simulink model "water_4hopper_VDF"  (Simulink 8.0)
settings: Solver=ode23t  StartTime=0.0  StopTime=5  MaxStep=1e-2  RelTol=1e-6
values from neighbouring files (symbols this model uses):
  alpha = 30    [SimParam_4VDF.m]
  amp = leg_length    (= 0.0249)    [SimParam_4VDF.m]
  C_d = 0.703    [SimParam_4VDF.m]
  density = 1000    [SimParam_4VDF.m]
  frame_inertia = diag([Ix,Iy,Iz])    [SimParam_4VDF.m]
  freq = 60    [SimParam_4VDF.m]
  g = 9.81    [SimParam_4VDF.m]
  K_d = 0    [SimParam_4VDF.m]
  K_i = 0    [SimParam_4VDF.m]
  K_p = -50    [SimParam_4VDF.m]
  leg_length = 0.0249    [SimParam_4VDF.m]
  m_toe = 0.0    (= 0)    [SimParam_4VDF.m]
  mass = 0.1    [SimParam_4VDF.m]
  S1 = pi*r1^2*0.9185    (= 0.00115422114093)    [SimParam_4VDF.m]
  S2 = pi*r2^2*0.9185    (= 7.21388213081e-05)    [SimParam_4VDF.m]
  tau = 0.001    [SimParam_4VDF.m]
undefined symbols (not defined in the file): y_0
libraries: mblibv1 x48, powerlib_extras x4, simulink x2
(part 1 of 2)
settings Model: Creator=Metti  LastModifiedBy=Metti
settings SolverCC: ZeroCrossControl=DisableAll
settings DataIOCC: SignalLoggingSaveFormat=ModelDataLogs
settings DebuggingCC: FcnCallInpInsideContextMsg=EnableAllAsWarning
settings SimMechanicsCC: VisOnUpdateDiagram=on  VisDuringSimulation=on  VisSampleTime=0.05  AutoFitVis=GROWTOFIT  LastVizWinPosition=[520 378 560 420]  CamPosition=[0;0;11.3949;]  CamTarget=[0;0;0;]  CamUpVector=[0;1;0;]  CamHeight=0.51  VisBackgroundColor=[0.9;0.9;0.95;]  DefaultBodyColor=[1;0;0;]
settings ConfigurationSet: Description=SimMechanics 2G

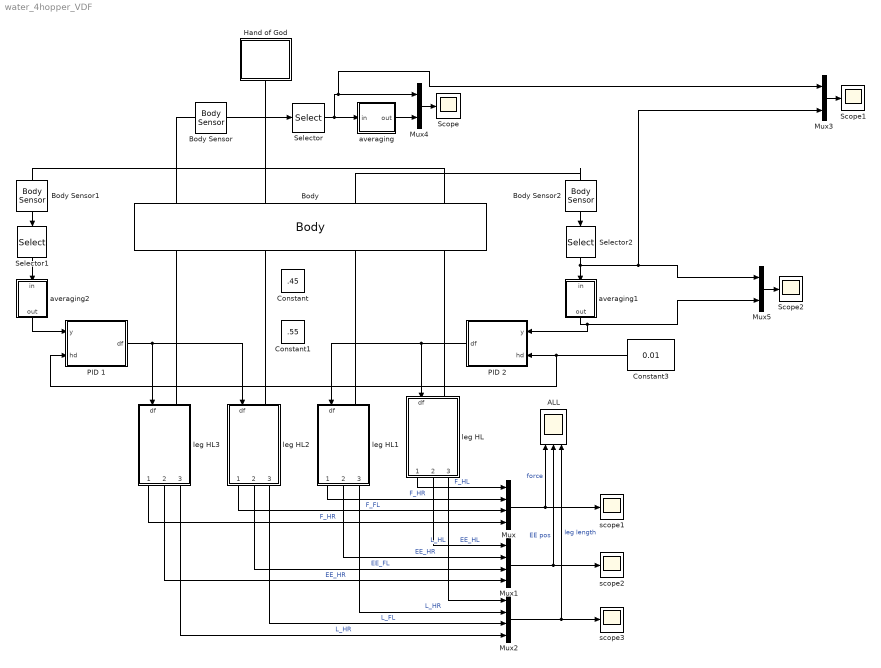
== system water_4hopper_VDF ==
  ALL : Scope  NumInputPorts=3
      settings: ShowLegends=on  TimeRange=10  YMin=-1~-50~-0.06  YMax=7~200~0.06  SaveName=ScopeData4
  Body : mblibv1/Bodies/Body  LConnTagsString=CG|CS1|CS6|CS7  RConnTagsString=CS2|CS3|CS4|CS5  UpdateFromCAD=off  DialogClass=MechanicalBodyBlock  Mass=mass  MassUnits=kg  InertiaUnits=kg*m^2  Inertia=frame_inertia  Shape=Cylinder  ShapeDims=[1 1]  ShapeUnits=m  ShapeUse=false  Density=1  DensityUnits=kg/m^3  DensityUse=false  GraphicsMode=MACHINE_DEFAULT  BodyColorSelMode=MACHINE_DEFAULT  BodyColor=[1 0 0]  AttachedToCS=CG  CG=Left$CG$CG_pos$CS1$CS1$m$[0 0 0]$Euler X-Y-Z$deg$WORLD$true$none  WorkingFrames=Left$CS1$[0 0 0]$Adjoining$Adjoining$m$[0 0 0]$Euler X-Y-Z$deg$WORLD$true$none#Right$CS2$TR_FR$CS1$CS1$m$[0 0 0]$Euler X-Y-Z$deg$WORLD$true$none#Right$CS3$TR_FL$CS1$CS1$m$[0 0 0]$Euler X-Y-Z$deg$WORLD$true$none#Right$CS4$TR_HR$CS1$CS1$m$[0 0 0]$Euler X-Y-Z$deg$WORLD$true$none#Right$CS5$TR_HL$CS1$CS1$m$[0 0 0]$Euler X-Y-Z$deg$WORLD$true$none#Left$CS6$TR_HL$CS1$CS1$m$[0 0 0]$Euler X-Y-Z$deg$WORLD$true$none#Left$CS7$TR_FR$CS1$CS1$m$[0 0 0]$Euler X-Y-Z$deg$WORLD$true$none  CGPos=CG_pos  CGRot=[0 0 0]  CS0Pos=[]  CS0Rot=[]  CS1Pos=[0 0 0]  CS1Rot=[0 0 0]  CS2Pos=TR_FR  CS2Rot=[0 0 0]  CS3Pos=TR_FL  CS3Rot=[0 0 0]  CS4Pos=TR_HR  CS4Rot=[0 0 0]  CS5Pos=TR_HL  CS5Rot=[0 0 0]  CS6Pos=TR_HL  CS6Rot=[0 0 0]  CS7Pos=TR_FR  CS7Rot=[0 0 0]  CS8Pos=[]  CS8Rot=[]  CS9Pos=[]  CS9Rot=[]  CS10Pos=[]  CS10Rot=[]  CS11Pos=[]  CS11Rot=[]  CS12Pos=[]  CS12Rot=[]  CS13Pos=[]  CS13Rot=[]  CS14Pos=[]  CS14Rot=[]  CS15Pos=[]  CS15Rot=[]  CS16Pos=[]  CS16Rot=[]  CS17Pos=[]  CS17Rot=[]  CS18Pos=[]  CS18Rot=[]  CS19Pos=[]  CS19Rot=[]  CS20Pos=[]  CS20Rot=[]
  Body Sensor : mblibv1/Sensors &  Actuators/Body Sensor  UpdateFromCAD=off  PhysicalDomain=Mechanical  PortType=blob  Muxed=on  Pose=off  Angle=on  AngleUnits=deg  ArcVelocity=off  ArcVelocityUnits=deg/s  ArcAcceleration=off  ArcAccelerationUnits=deg/s^2  CoordPosition=on  CoordPositionUnits=m  Velocity=off  VelocityUnits=m/s  Acceleration=off  AccelerationUnits=m/s^2  Quaternion=on  QuaternionDT=off  QuaternionDDT=off  QuaternionUnits=off  OutputVector=[1]  ActiveIO=on  Width=3  DialogClass=MechanicalSensorBlock  ReferenceFrame=Absolute (World)
  Body Sensor1 : mblibv1/Sensors &  Actuators/Body Sensor  UpdateFromCAD=off  PhysicalDomain=Mechanical  PortType=blob  Muxed=on  Pose=off  Angle=on  AngleUnits=deg  ArcVelocity=off  ArcVelocityUnits=deg/s  ArcAcceleration=off  ArcAccelerationUnits=deg/s^2  CoordPosition=on  CoordPositionUnits=m  Velocity=off  VelocityUnits=m/s  Acceleration=off  AccelerationUnits=m/s^2  Quaternion=on  QuaternionDT=off  QuaternionDDT=off  QuaternionUnits=off  OutputVector=[1]  ActiveIO=on  Width=3  DialogClass=MechanicalSensorBlock  ReferenceFrame=Absolute (World)
  Body Sensor2 : mblibv1/Sensors &  Actuators/Body Sensor  UpdateFromCAD=off  PhysicalDomain=Mechanical  PortType=blob  Muxed=on  Pose=off  Angle=on  AngleUnits=deg  ArcVelocity=off  ArcVelocityUnits=deg/s  ArcAcceleration=off  ArcAccelerationUnits=deg/s^2  CoordPosition=on  CoordPositionUnits=m  Velocity=off  VelocityUnits=m/s  Acceleration=off  AccelerationUnits=m/s^2  Quaternion=on  QuaternionDT=off  QuaternionDDT=off  QuaternionUnits=off  OutputVector=[1]  ActiveIO=on  Width=3  DialogClass=MechanicalSensorBlock  ReferenceFrame=Absolute (World)
  Constant : Constant  Value=.45
  Constant1 : Constant  Value=.55
  Constant3 : Constant  Value=0.01
  Hand of God : Subsystem
  Mux : Mux
  Mux1 : Mux
  Mux2 : Mux
  Mux3 : Mux  Inputs=2
  Mux4 : Mux  Inputs=2
  Mux5 : Mux  Inputs=2
  PID 1 : Subsystem
  PID 2 : Subsystem
  Scope : Scope
      settings: TimeRange=5  YMin=-0.025  YMax=0.02
  Scope1 : Scope
      settings: YMin=0.0915  YMax=0.09575  SaveName=ScopeData5
  Scope2 : Scope
      settings: YMin=0.0915  YMax=0.09575  SaveName=ScopeData12
  Selector : Selector  InputPortWidth=3  IndexOptions=Index vector (dialog)  Indices=[2]  OutputSizes=1
  Selector1 : Selector  InputPortWidth=3  IndexOptions=Index vector (dialog)  Indices=[2]  OutputSizes=1
  Selector2 : Selector  InputPortWidth=3  IndexOptions=Index vector (dialog)  Indices=[2]  OutputSizes=1
  averaging : Subsystem  mask{T_win=2*pi/freq/2, x_init=y_0}
      mask prompts: T_win "window (s)"; x_init "Initial condition"
  averaging1 : Subsystem  mask{T_win=2*pi/freq, x_init=y_0}
      mask prompts: T_win "window (s)"; x_init "Initial condition"
  averaging2 : Subsystem  mask{T_win=2*pi/freq, x_init=y_0}
      mask prompts: T_win "window (s)"; x_init "Initial condition"
  leg HL : Subsystem
  leg HL1 : Subsystem
  leg HL2 : Subsystem
  leg HL3 : Subsystem
  "scope1 " : Scope
      settings: ShowLegends=on
  scope2 : Scope
      settings: ShowLegends=on  SaveName=ScopeData2
  scope3 : Scope
      settings: ShowLegends=on  SaveName=ScopeData3
  wires:
  Body Sensor/1 -> Selector/1
  Mux/1 -> "scope1 "/1, ALL/1  "force"
  leg HL/1(force) -> Mux/1  "F_HL"
  leg HL1/1(force) -> Mux/2  "F_HR"
  leg HL2/1(force) -> Mux/3  "F_FL"
  leg HL3/1(force) -> Mux/4  "F_HR"
  Mux1/1 -> ALL/2, scope2/1  "EE pos"
  leg HL/2(EE pos) -> Mux1/1  "EE_HL"
  leg HL1/2(EE pos) -> Mux1/2  "EE_HR"
  leg HL3/2(EE pos) -> Mux1/4  "EE_HR"
  leg HL2/2(EE pos) -> Mux1/3  "EE_FL"
  Mux2/1 -> ALL/3, scope3/1  "leg length"
  leg HL/3(leg length) -> Mux2/1  "L_HL"
  leg HL1/3(leg length) -> Mux2/2  "L_HR"
  leg HL2/3(leg length) -> Mux2/3  "L_FL"
  leg HL3/3(leg length) -> Mux2/4  "L_HR"
  averaging/1(out) -> Mux4/2
  Mux4/1 -> Scope/1
  Body Sensor1/1 -> Selector1/1
  Body Sensor2/1 -> Selector2/1
  Selector2/1 -> averaging1/1(in), Mux3/2, Mux5/1
  Constant3/1 -> PID 1/2(hd), PID 2/2(hd)
  Selector1/1 -> averaging2/1(in)
  Mux5/1 -> Scope2/1
  averaging1/1(out) -> PID 2/1(y), Mux5/2
  averaging2/1(out) -> PID 1/1(y)
  PID 2/1(df) -> leg HL1/1(df), leg HL/1(df)
  PID 1/1(df) -> leg HL3/1(df), leg HL2/1(df)
  Mux3/1 -> Scope1/1
  Selector/1 -> averaging/1(in), Mux3/1, Mux4/1
  connections:
  Hand of God/RConn1 -- Body/LConn2
  leg HL2/LConn1 -- Body/RConn2
  leg HL1/LConn1 -- Body/RConn3
  Body/RConn4 -- leg HL/LConn1
  leg HL3/LConn1 -- Body/RConn1
  Body Sensor1/LConn1 -- Body/LConn4
  Body Sensor2/LConn1 -- Body/LConn3
  Body Sensor/LConn1 -- Body/LConn1

== system water_4hopper_VDF/Hand of God ==
  Custom Joint : mblibv1/Joints/Custom Joint  LConnTagsString=__newl0|SA1  RConnTagsString=__newr0  UpdateFromCAD=off  NumSAPorts=1  CutJoint=off  MarkAsCut=off  Primitives=prismatic  PrimitiveProps=P1$World$[0 1 0]$Prismatic#P2$World$[1 0 0]$Prismatic#R1$World$[1 0 0]$Revolute#R2$World$[0 0 1]$Revolute  DialogClass=JointBlock  R1Axis=[1 0 0]  R2Axis=[0 0 1]  R3Axis=[]  P1Axis=[0 1 0]  P2Axis=[1 0 0]  P3Axis=[]  SAxis=[]
  Ground : mblibv1/Bodies/Ground  UpdateFromCAD=off  LeftPortType=env  RightPortType=workingframe  PhysicalDomain=Mechanical  DialogClass=GroundBlock  CoordPosition=[0 0 0]  CoordPositionUnits=m  StateVectorMgrId=0  MachineId=[1 0]  ShowEnvPort=on
  Joint Initial Condition : mblibv1/Sensors &  Actuators/Joint Initial Condition  UpdateFromCAD=off  LeftPortType=blob  RightPortType=blob  PhysicalDomain=mechanical  DialogClass=InitialConditionBlock  InitialConditions=P1$true$y_0$m$deg$0$m/s$deg/s#P2$false$y_0$m$deg$0$m/s$deg/s#P3$false$0$m$deg$0$m/s$deg/s#R1$true$0$m$deg$0$m/s$deg/s#R2$true$0$m$deg$0$m/s$deg/s#R3$false$10$m$deg$0$m/s$deg/s#S$false$0$m$deg$0$m/s$deg/s  P1PIC=y_0  P1VIC=0  P2PIC=0  P2VIC=0  P3PIC=0  P3VIC=0  R1PIC=0  R1VIC=0  R2PIC=0  R2VIC=0  R3PIC=0  R3VIC=0  SPIC=0  SVIC=0
  Joint Sensor : mblibv1/Sensors &  Actuators/Joint Sensor  UpdateFromCAD=off  PhysicalDomain=Mechanical  PortType=blob  Muxed=on  Pose=off  Angle=on  AngleUnits=deg  ArcVelocity=off  ArcVelocityUnits=deg/s  ArcAcceleration=off  ArcAccelerationUnits=deg/s^2  CoordPosition=on  CoordPositionUnits=m  Velocity=off  VelocityUnits=m/s  Acceleration=off  AccelerationUnits=m/s^2  Quaternion=on  QuaternionDT=off  QuaternionDDT=off  QuaternionUnits=off  OutputVector=[1]  ActiveIO=on  Width=1  DialogClass=MechanicalSensorBlock  Primitive=P1  Force=off  ForceUnits=N  Torque=off  TorqueUnits=N*m  ReferenceFrame=Absolute (World)  ReactionSensedSide=Base  ReactionReferenceFrame=Absolute (World)  ReactionForce=off  ReactionForceUnits=N  ReactionMoment=off  ReactionMomentUnits=N*m
  Joint Sensor1 : mblibv1/Sensors &  Actuators/Joint Sensor  UpdateFromCAD=off  PhysicalDomain=Mechanical  PortType=blob  Muxed=on  Pose=off  Angle=on  AngleUnits=deg  ArcVelocity=off  ArcVelocityUnits=deg/s  ArcAcceleration=off  ArcAccelerationUnits=deg/s^2  CoordPosition=on  CoordPositionUnits=m  Velocity=off  VelocityUnits=m/s  Acceleration=off  AccelerationUnits=m/s^2  Quaternion=on  QuaternionDT=off  QuaternionDDT=off  QuaternionUnits=off  OutputVector=[1]  ActiveIO=on  Width=1  DialogClass=MechanicalSensorBlock  Primitive=R1  Force=off  ForceUnits=N  Torque=off  TorqueUnits=N*m  ReferenceFrame=Absolute (World)  ReactionSensedSide=Base  ReactionReferenceFrame=Absolute (World)  ReactionForce=off  ReactionForceUnits=N  ReactionMoment=off  ReactionMomentUnits=N*m
  Joint Sensor2 : mblibv1/Sensors &  Actuators/Joint Sensor  UpdateFromCAD=off  PhysicalDomain=Mechanical  PortType=blob  Muxed=off  Pose=off  Angle=on  AngleUnits=deg  ArcVelocity=off  ArcVelocityUnits=deg/s  ArcAcceleration=off  ArcAccelerationUnits=deg/s^2  CoordPosition=on  CoordPositionUnits=m  Velocity=off  VelocityUnits=m/s  Acceleration=off  AccelerationUnits=m/s^2  Quaternion=on  QuaternionDT=off  QuaternionDDT=off  QuaternionUnits=off  OutputVector=[1]  ActiveIO=on  Width=1  DialogClass=MechanicalSensorBlock  Primitive=R2  Force=off  ForceUnits=N  Torque=off  TorqueUnits=N*m  ReferenceFrame=Absolute (World)  ReactionSensedSide=Base  ReactionReferenceFrame=Absolute (World)  ReactionForce=off  ReactionForceUnits=N  ReactionMoment=off  ReactionMomentUnits=N*m
  Machine Environment : mblibv1/Bodies/Machine Environment  PortType=env  PhysicalDomain=Mechanical  DialogTemplateClass=MECH.MachineEnvironment  SyncWhenCopied=off  Gravity=[0 -g 0]  GravityUnits=m/s^2  GravityAsSignal=off  Dimensionality=Auto-detect  AnalysisType=Forward dynamics  LinearAssemblyTolerance=1e-3  LinearAssemblyToleranceUnits=m  AngularAssemblyTolerance=1e-3  AngularAssemblyToleranceUnits=rad  ConstraintSolverType=Stabilizing  ConstraintRelTolerance=1e-4  ConstraintAbsTolerance=1e-4  UseRobustSingularityHandling=off  RedundancyAnalysisToleranceType=Automatically select tolerance  RedundancyAnalysisTolerance=1e-14  StatePerturbationType=Fixed  PerturbationSize=1e-5  VisualizeMachine=on  BodyVisualizationType=Use model default body geometries  BodyColorSelMode=Use model default  DefaultBodyColor=[1 0 0]
  Mechanical Branching Bar : mblibv1/Utilities/Mechanical Branching Bar  LConnTagsString=_newl0  RConnTagsString=__newr0|SA2|SA3|SA4  UpdateFromCAD=off  DialogClass=MechanicalBranchingBarBlock  NumSAPorts=4
  Scope : Scope  NumInputPorts=3
      settings: TimeRange=5  YMin=-0.01~-0.001~-6  YMax=0.02~0.0004~1  SaveName=mass_data
  Conn1 : PMIOPort  Port=1  Side=Right
  wires:
  Joint Sensor/1 -> Scope/1
  Joint Sensor1/1 -> Scope/2
  Joint Sensor2/1 -> Scope/3
  connections:
  Conn1/RConn1 -- Custom Joint/RConn1
  Joint Sensor1/LConn1 -- Mechanical Branching Bar/RConn3
  Ground/RConn1 -- Custom Joint/LConn1
  Machine Environment/RConn1 -- Ground/LConn1
  Joint Initial Condition/RConn1 -- Mechanical Branching Bar/RConn1
  Joint Sensor/LConn1 -- Mechanical Branching Bar/RConn2
  Custom Joint/LConn2 -- Mechanical Branching Bar/LConn1
  Joint Sensor2/LConn1 -- Mechanical Branching Bar/RConn4

== system water_4hopper_VDF/PID 1 ==
  y : Inport
  hd : Inport  Port=2
  Constant : Constant  Value=.55
  Fcn : Fcn  Expr=u(1)^2
  Fcn1 : Fcn  Expr=u(1)^2
  Gain3 : Gain
  Mux4 : Mux  Inputs=2
  PID Controller : simulink/Continuous/PID Controller  Controller=PID  TimeDomain=Continuous-time  SampleTime=1  IntegratorMethod=Forward Euler  FilterMethod=Forward Euler  Form=Parallel  P=K_p  I=K_i  D=K_d  N=100  InitialConditionSource=internal  InitialConditionForIntegrator=0  InitialConditionForFilter=0  ExternalReset=none  LimitOutput=off  UpperSaturationLimit=inf  LowerSaturationLimit=-inf  LinearizeAsGain=on  AntiWindupMode=none  Kb=1  TrackingMode=off  Kt=1  PParamMin=[]  PParamMax=[]  IParamMin=[]  IParamMax=[]  DParamMin=[]  DParamMax=[]  NParamMin=[]  NParamMax=[]  KbParamMin=[]  KbParamMax=[]  KtParamMin=[]  KtParamMax=[]  POutMin=[]  POutMax=[]  IOutMin=[]  IOutMax=[]  DOutMin=[]  DOutMax=[]  NOutMin=[]  NOutMax=[]  KbOutMin=[]  KbOutMax=[]  KtOutMin=[]  KtOutMax=[]  IntegratorOutMin=[]  IntegratorOutMax=[]  FilterOutMin=[]  FilterOutMax=[]  SumOutMin=[]  SumOutMax=[]  SumI1OutMin=[]  SumI1OutMax=[]  SumI2OutMin=[]  SumI2OutMax=[]  SumI3OutMin=[]  SumI3OutMax=[]  SumDOutMin=[]  SumDOutMax=[]  SaturationOutMin=[]  SaturationOutMax=[]  IntegratorContinuousStateAttributes=''  IntegratorStateMustResolveToSignalObject=off  IntegratorRTWStateStorageClass=Auto  FilterContinuousStateAttributes=''  FilterStateMustResolveToSignalObject=off  FilterRTWStateStorageClass=Auto
  Saturation2 : Saturate  UpperLimit=0.7  LowerLimit=0.3
  Scope1 : Scope  NumInputPorts=2
      settings: TimeRange=5  YMin=0.0575~-0.0125  YMax=0.0875~0.015
  Scope3 : Scope
      settings: SaveName=ScopeData4
  Sum3 : Sum  Inputs=|+-
  Sum4 : Sum  Inputs=|-+
  df : Outport
  wires:
  PID Controller/1 -> Gain3/1
  Sum3/1 -> PID Controller/1, Scope1/2
  Gain3/1 -> Sum4/1
  Mux4/1 -> Scope1/1
  y/1 -> Fcn1/1, Mux4/2
  hd/1 -> Mux4/1, Fcn/1
  Sum4/1 -> Saturation2/1
  Saturation2/1 -> Scope3/1, df/1
  Constant/1 -> Sum4/2
  Fcn/1 -> Sum3/1
  Fcn1/1 -> Sum3/2

== system water_4hopper_VDF/PID 2 ==
  y : Inport
  hd : Inport  Port=2
  Constant : Constant  Value=.45
  Fcn : Fcn  Expr=u(1)^2
  Fcn1 : Fcn  Expr=u(1)^2
  Gain3 : Gain
  Mux4 : Mux  Inputs=2
  PID Controller : simulink/Continuous/PID Controller  Controller=PID  TimeDomain=Continuous-time  SampleTime=1  IntegratorMethod=Forward Euler  FilterMethod=Forward Euler  Form=Parallel  P=K_p  I=K_i  D=K_d  N=100  InitialConditionSource=internal  InitialConditionForIntegrator=0  InitialConditionForFilter=0  ExternalReset=none  LimitOutput=off  UpperSaturationLimit=inf  LowerSaturationLimit=-inf  LinearizeAsGain=on  AntiWindupMode=none  Kb=1  TrackingMode=off  Kt=1  PParamMin=[]  PParamMax=[]  IParamMin=[]  IParamMax=[]  DParamMin=[]  DParamMax=[]  NParamMin=[]  NParamMax=[]  KbParamMin=[]  KbParamMax=[]  KtParamMin=[]  KtParamMax=[]  POutMin=[]  POutMax=[]  IOutMin=[]  IOutMax=[]  DOutMin=[]  DOutMax=[]  NOutMin=[]  NOutMax=[]  KbOutMin=[]  KbOutMax=[]  KtOutMin=[]  KtOutMax=[]  IntegratorOutMin=[]  IntegratorOutMax=[]  FilterOutMin=[]  FilterOutMax=[]  SumOutMin=[]  SumOutMax=[]  SumI1OutMin=[]  SumI1OutMax=[]  SumI2OutMin=[]  SumI2OutMax=[]  SumI3OutMin=[]  SumI3OutMax=[]  SumDOutMin=[]  SumDOutMax=[]  SaturationOutMin=[]  SaturationOutMax=[]  IntegratorContinuousStateAttributes=''  IntegratorStateMustResolveToSignalObject=off  IntegratorRTWStateStorageClass=Auto  FilterContinuousStateAttributes=''  FilterStateMustResolveToSignalObject=off  FilterRTWStateStorageClass=Auto
  Saturation2 : Saturate  UpperLimit=0.7  LowerLimit=0.3
  Scope1 : Scope  NumInputPorts=2
      settings: TimeRange=5  YMin=0.0575~-0.0125  YMax=0.0875~0.015
  Scope3 : Scope
      settings: SaveName=ScopeData4
  Sum3 : Sum  Inputs=|+-
  Sum4 : Sum  Inputs=|-+
  df : Outport
  wires:
  PID Controller/1 -> Gain3/1
  Sum3/1 -> Scope1/2, PID Controller/1
  Gain3/1 -> Sum4/1
  Mux4/1 -> Scope1/1
  Sum4/1 -> Saturation2/1
  Constant/1 -> Sum4/2
  Fcn/1 -> Sum3/1
  Fcn1/1 -> Sum3/2
  y/1 -> Fcn1/1, Mux4/2
  hd/1 -> Mux4/1, Fcn/1
  Saturation2/1 -> Scope3/1, df/1

== system water_4hopper_VDF/averaging ==
  in : Inport
  Constant1 : Constant  Value=x_init
  Gain : Gain  Gain=1/T_win
  Integrator1 : Integrator
  Sum : Sum  Inputs=+-|
  Sum1 : Sum  Inputs=-+|
  Sum3 : Sum  Inputs=++|
  Transport Delay : TransportDelay  DelayTime=T_win
  out : Outport
  wires:
  in/1 -> Sum1/2
  Gain/1 -> Sum3/2
  Constant1/1 -> Sum3/1, Sum1/1
  Sum1/1 -> Integrator1/1
  Transport Delay/1 -> Sum/2
  Integrator1/1 -> Sum/1, Transport Delay/1
  Sum3/1 -> out/1
  Sum/1 -> Gain/1

== system water_4hopper_VDF/averaging1 ==
  in : Inport
  Constant1 : Constant  Value=x_init
  Gain : Gain  Gain=1/T_win
  Integrator1 : Integrator
  Sum : Sum  Inputs=+-|
  Sum1 : Sum  Inputs=-+|
  Sum3 : Sum  Inputs=++|
  Transport Delay : TransportDelay  DelayTime=T_win
  out : Outport
  wires:
  in/1 -> Sum1/2
  Gain/1 -> Sum3/2
  Constant1/1 -> Sum3/1, Sum1/1
  Sum1/1 -> Integrator1/1
  Transport Delay/1 -> Sum/2
  Integrator1/1 -> Sum/1, Transport Delay/1
  Sum3/1 -> out/1
  Sum/1 -> Gain/1

== system water_4hopper_VDF/averaging2 ==
  in : Inport
  Constant1 : Constant  Value=x_init
  Gain : Gain  Gain=1/T_win
  Integrator1 : Integrator
  Sum : Sum  Inputs=+-|
  Sum1 : Sum  Inputs=-+|
  Sum3 : Sum  Inputs=++|
  Transport Delay : TransportDelay  DelayTime=T_win
  out : Outport
  wires:
  Sum/1 -> Gain/1
  Sum3/1 -> out/1
  Integrator1/1 -> Transport Delay/1, Sum/1
  Transport Delay/1 -> Sum/2
  Sum1/1 -> Integrator1/1
  Constant1/1 -> Sum1/1, Sum3/1
  Gain/1 -> Sum3/2
  in/1 -> Sum1/2

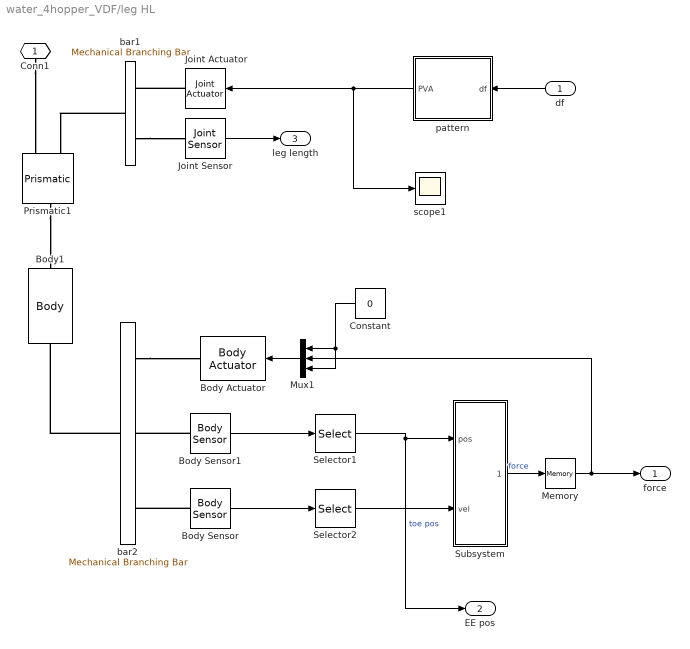
== system water_4hopper_VDF/leg HL ==
  df : Inport
  Body Actuator : mblibv1/Sensors &  Actuators/Body Actuator  UpdateFromCAD=off  PhysicalDomain=Mechanical  PortType=blob  ActuationStyle=Force  AngleUnits=deg  ArcVelocityUnits=deg/s  ArcAccelerationUnits=deg/s^2  CoordPositionUnits=m  VelocityUnits=m/s  AccelerationUnits=m/s^2  ForceUnits=N  TorqueUnits=N*m  ActiveIO=on  Width=3  DialogClass=MechanicalActuatorBlock  ReferenceFrame=Local (Body CS)  Angle=off  CoordPosition=on  Force=on  Torque=off
  Body Sensor : mblibv1/Sensors &  Actuators/Body Sensor  UpdateFromCAD=off  PhysicalDomain=Mechanical  PortType=blob  Muxed=on  Pose=off  Angle=on  AngleUnits=deg  ArcVelocity=off  ArcVelocityUnits=deg/s  ArcAcceleration=off  ArcAccelerationUnits=deg/s^2  CoordPosition=off  CoordPositionUnits=m  Velocity=on  VelocityUnits=m/s  Acceleration=off  AccelerationUnits=m/s^2  Quaternion=on  QuaternionDT=off  QuaternionDDT=off  QuaternionUnits=off  OutputVector=[1]  ActiveIO=on  Width=3  DialogClass=MechanicalSensorBlock  ReferenceFrame=Local (Body CS)
  Body Sensor1 : mblibv1/Sensors &  Actuators/Body Sensor  UpdateFromCAD=off  PhysicalDomain=Mechanical  PortType=blob  Muxed=on  Pose=off  Angle=on  AngleUnits=deg  ArcVelocity=off  ArcVelocityUnits=deg/s  ArcAcceleration=off  ArcAccelerationUnits=deg/s^2  CoordPosition=on  CoordPositionUnits=m  Velocity=off  VelocityUnits=m/s  Acceleration=off  AccelerationUnits=m/s^2  Quaternion=on  QuaternionDT=off  QuaternionDDT=off  QuaternionUnits=off  OutputVector=[1]  ActiveIO=on  Width=3  DialogClass=MechanicalSensorBlock  ReferenceFrame=Absolute (World)
  Body1 : mblibv1/Bodies/Body  LConnTagsString=CG  RConnTagsString=CS1  UpdateFromCAD=off  DialogClass=MechanicalBodyBlock  Mass=m_toe  MassUnits=kg  InertiaUnits=kg*m^2  Inertia=0.*eye(3)  Shape=Cylinder  ShapeDims=[1 1]  ShapeUnits=m  ShapeUse=false  Density=1  DensityUnits=kg/m^3  DensityUse=false  GraphicsMode=CONVHULL  BodyColorSelMode=MACHINE_DEFAULT  BodyColor=[1 0 0]  AttachedToCS=CG  CG=Left$CG$[0 0 0]$Adjoining$Adjoining$m$[0 0 0]$Euler X-Y-Z$deg$WORLD$true$none  WorkingFrames=Right$CS1$[0 -leg_length 0]$CG$CG$m$[0 0 0]$Euler X-Y-Z$deg$WORLD$true$none#Left$CS2$[0 0 0]$CG$CG$m$[0 0 0]$Euler X-Y-Z$deg$WORLD$false$none  CGPos=[0 0 0]  CGRot=[0 0 0]  CS0Pos=[]  CS0Rot=[]  CS1Pos=[0 -leg_length 0]  CS1Rot=[0 0 0]  CS2Pos=[0 0 0]  CS2Rot=[0 0 0]  CS3Pos=[]  CS3Rot=[]  CS4Pos=[]  CS4Rot=[]  CS5Pos=[]  CS5Rot=[]  CS6Pos=[]  CS6Rot=[]  CS7Pos=[]  CS7Rot=[]  CS8Pos=[]  CS8Rot=[]  CS9Pos=[]  CS9Rot=[]  CS10Pos=[]  CS10Rot=[]  CS11Pos=[]  CS11Rot=[]  CS12Pos=[]  CS12Rot=[]  CS13Pos=[]  CS13Rot=[]  CS14Pos=[]  CS14Rot=[]  CS15Pos=[]  CS15Rot=[]  CS16Pos=[]  CS16Rot=[]  CS17Pos=[]  CS17Rot=[]  CS18Pos=[]  CS18Rot=[]  CS19Pos=[]  CS19Rot=[]  CS20Pos=[]  CS20Rot=[]
  Constant : Constant  Value=0
  Joint Actuator : mblibv1/Sensors &  Actuators/Joint Actuator  UpdateFromCAD=off  PhysicalDomain=Mechanical  PortType=blob  ActuationStyle=Motion  AngleUnits=deg  ArcVelocityUnits=deg/s  ArcAccelerationUnits=deg/s^2  CoordPositionUnits=m  VelocityUnits=m/s  AccelerationUnits=m/s^2  ForceUnits=N  TorqueUnits=N*m  ActiveIO=on  Width=3  DialogClass=MechanicalActuatorBlock  Primitive=P1  ReferenceFrame=Absolute (World)
  Joint Sensor : mblibv1/Sensors &  Actuators/Joint Sensor  UpdateFromCAD=off  PhysicalDomain=Mechanical  PortType=blob  Muxed=on  Pose=off  Angle=on  AngleUnits=deg  ArcVelocity=off  ArcVelocityUnits=deg/s  ArcAcceleration=off  ArcAccelerationUnits=deg/s^2  CoordPosition=on  CoordPositionUnits=m  Velocity=off  VelocityUnits=m/s  Acceleration=off  AccelerationUnits=m/s^2  Quaternion=on  QuaternionDT=off  QuaternionDDT=off  QuaternionUnits=off  OutputVector=[1]  ActiveIO=on  Width=1  DialogClass=MechanicalSensorBlock  Primitive=P1  Force=off  ForceUnits=N  Torque=off  TorqueUnits=N*m  ReferenceFrame=Absolute (World)  ReactionSensedSide=Base  ReactionReferenceFrame=Absolute (World)  ReactionForce=off  ReactionForceUnits=N  ReactionMoment=off  ReactionMomentUnits=N*m
  Memory : Memory
  Mux1 : Mux  Inputs=3
  Prismatic1 : mblibv1/Joints/Prismatic  LConnTagsString=__newl0|SA1  RConnTagsString=__newr0  UpdateFromCAD=off  NumSAPorts=1  CutJoint=off  MarkAsCut=off  Primitives=prismatic  PrimitiveProps=P1$World$[0 1 0]$prismatic  DialogClass=JointBlock  P1Axis=[0 1 0]
  Selector1 : Selector  InputPortWidth=3  IndexOptions=Index vector (dialog)  Indices=[2]  OutputSizes=1
  Selector2 : Selector  InputPortWidth=3  IndexOptions=Index vector (dialog)  Indices=[2]  OutputSizes=1
  Subsystem : Subsystem
  bar1 : mblibv1/Utilities/Mechanical Branching Bar  LConnTagsString=_newl0  RConnTagsString=SA0|SA1  UpdateFromCAD=off  DialogClass=MechanicalBranchingBarBlock  NumSAPorts=2
  bar2 : mblibv1/Utilities/Mechanical Branching Bar  LConnTagsString=_newl0  RConnTagsString=__newr0|SA2|SA3  UpdateFromCAD=off  DialogClass=MechanicalBranchingBarBlock  NumSAPorts=3
  pattern : Subsystem  mask{Amp=amp, Offset=0, freq=freq}
      mask prompts: Amp "Amplitude"; freq "Frequency"
      mask TypeOptions freq: Constant/Value
  "scope1 " : Scope
      settings: ShowLegends=on  SaveName=ScopeData11
  Conn1 : PMIOPort  Port=1  Side=Left
  force : Outport
  EE pos : Outport  Port=2
  leg length : Outport  Port=3
  wires:
  Mux1/1 -> Body Actuator/1
  Selector1/1 -> EE pos/1, Subsystem/1(pos)  "toe pos"
  Body Sensor/1 -> Selector2/1
  Joint Sensor/1 -> leg length/1
  Body Sensor1/1 -> Selector1/1
  Selector2/1 -> Subsystem/2(vel)
  Subsystem/1(force) -> Memory/1  "force"
  Constant/1 -> Mux1/1, Mux1/3
  df/1 -> pattern/1(df)
  pattern/1(PVA) -> "scope1 "/1, Joint Actuator/1
  Memory/1 -> Mux1/2, force/1
  connections:
  Conn1/RConn1 -- Prismatic1/LConn1
  bar2/LConn1 -- Body1/RConn1
  Prismatic1/RConn1 -- Body1/LConn1
  bar1/LConn1 -- Prismatic1/LConn2
  Joint Actuator/RConn1 -- bar1/RConn1
  bar1/RConn2 -- Joint Sensor/LConn1
  bar2/RConn1 -- Body Actuator/RConn1
  Body Sensor/LConn1 -- bar2/RConn3
  Body Sensor1/LConn1 -- bar2/RConn2

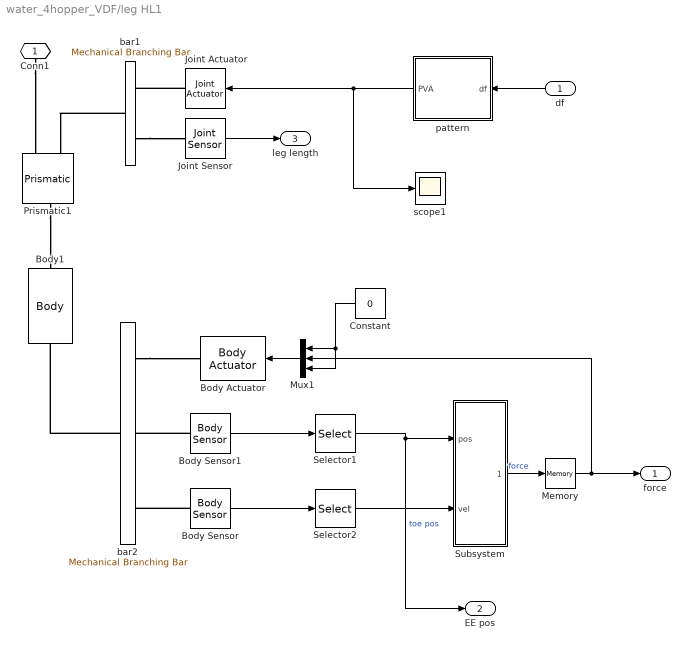
== system water_4hopper_VDF/leg HL1 ==
  df : Inport
  Body Actuator : mblibv1/Sensors &  Actuators/Body Actuator  UpdateFromCAD=off  PhysicalDomain=Mechanical  PortType=blob  ActuationStyle=Force  AngleUnits=deg  ArcVelocityUnits=deg/s  ArcAccelerationUnits=deg/s^2  CoordPositionUnits=m  VelocityUnits=m/s  AccelerationUnits=m/s^2  ForceUnits=N  TorqueUnits=N*m  ActiveIO=on  Width=3  DialogClass=MechanicalActuatorBlock  ReferenceFrame=Local (Body CS)  Angle=off  CoordPosition=on  Force=on  Torque=off
  Body Sensor : mblibv1/Sensors &  Actuators/Body Sensor  UpdateFromCAD=off  PhysicalDomain=Mechanical  PortType=blob  Muxed=on  Pose=off  Angle=on  AngleUnits=deg  ArcVelocity=off  ArcVelocityUnits=deg/s  ArcAcceleration=off  ArcAccelerationUnits=deg/s^2  CoordPosition=off  CoordPositionUnits=m  Velocity=on  VelocityUnits=m/s  Acceleration=off  AccelerationUnits=m/s^2  Quaternion=on  QuaternionDT=off  QuaternionDDT=off  QuaternionUnits=off  OutputVector=[1]  ActiveIO=on  Width=3  DialogClass=MechanicalSensorBlock  ReferenceFrame=Local (Body CS)
  Body Sensor1 : mblibv1/Sensors &  Actuators/Body Sensor  UpdateFromCAD=off  PhysicalDomain=Mechanical  PortType=blob  Muxed=on  Pose=off  Angle=on  AngleUnits=deg  ArcVelocity=off  ArcVelocityUnits=deg/s  ArcAcceleration=off  ArcAccelerationUnits=deg/s^2  CoordPosition=on  CoordPositionUnits=m  Velocity=off  VelocityUnits=m/s  Acceleration=off  AccelerationUnits=m/s^2  Quaternion=on  QuaternionDT=off  QuaternionDDT=off  QuaternionUnits=off  OutputVector=[1]  ActiveIO=on  Width=3  DialogClass=MechanicalSensorBlock  ReferenceFrame=Absolute (World)
  Body1 : mblibv1/Bodies/Body  LConnTagsString=CG  RConnTagsString=CS1  UpdateFromCAD=off  DialogClass=MechanicalBodyBlock  Mass=m_toe  MassUnits=kg  InertiaUnits=kg*m^2  Inertia=0.*eye(3)  Shape=Cylinder  ShapeDims=[1 1]  ShapeUnits=m  ShapeUse=false  Density=1  DensityUnits=kg/m^3  DensityUse=false  GraphicsMode=CONVHULL  BodyColorSelMode=MACHINE_DEFAULT  BodyColor=[1 0 0]  AttachedToCS=CG  CG=Left$CG$[0 0 0]$Adjoining$Adjoining$m$[0 0 0]$Euler X-Y-Z$deg$WORLD$true$none  WorkingFrames=Right$CS1$[0 -leg_length 0]$CG$CG$m$[0 0 0]$Euler X-Y-Z$deg$WORLD$true$none#Left$CS2$[0 0 0]$CG$CG$m$[0 0 0]$Euler X-Y-Z$deg$WORLD$false$none  CGPos=[0 0 0]  CGRot=[0 0 0]  CS0Pos=[]  CS0Rot=[]  CS1Pos=[0 -leg_length 0]  CS1Rot=[0 0 0]  CS2Pos=[0 0 0]  CS2Rot=[0 0 0]  CS3Pos=[]  CS3Rot=[]  CS4Pos=[]  CS4Rot=[]  CS5Pos=[]  CS5Rot=[]  CS6Pos=[]  CS6Rot=[]  CS7Pos=[]  CS7Rot=[]  CS8Pos=[]  CS8Rot=[]  CS9Pos=[]  CS9Rot=[]  CS10Pos=[]  CS10Rot=[]  CS11Pos=[]  CS11Rot=[]  CS12Pos=[]  CS12Rot=[]  CS13Pos=[]  CS13Rot=[]  CS14Pos=[]  CS14Rot=[]  CS15Pos=[]  CS15Rot=[]  CS16Pos=[]  CS16Rot=[]  CS17Pos=[]  CS17Rot=[]  CS18Pos=[]  CS18Rot=[]  CS19Pos=[]  CS19Rot=[]  CS20Pos=[]  CS20Rot=[]
  Constant : Constant  Value=0
  Joint Actuator : mblibv1/Sensors &  Actuators/Joint Actuator  UpdateFromCAD=off  PhysicalDomain=Mechanical  PortType=blob  ActuationStyle=Motion  AngleUnits=deg  ArcVelocityUnits=deg/s  ArcAccelerationUnits=deg/s^2  CoordPositionUnits=m  VelocityUnits=m/s  AccelerationUnits=m/s^2  ForceUnits=N  TorqueUnits=N*m  ActiveIO=on  Width=3  DialogClass=MechanicalActuatorBlock  Primitive=P1  ReferenceFrame=Absolute (World)
  Joint Sensor : mblibv1/Sensors &  Actuators/Joint Sensor  UpdateFromCAD=off  PhysicalDomain=Mechanical  PortType=blob  Muxed=on  Pose=off  Angle=on  AngleUnits=deg  ArcVelocity=off  ArcVelocityUnits=deg/s  ArcAcceleration=off  ArcAccelerationUnits=deg/s^2  CoordPosition=on  CoordPositionUnits=m  Velocity=off  VelocityUnits=m/s  Acceleration=off  AccelerationUnits=m/s^2  Quaternion=on  QuaternionDT=off  QuaternionDDT=off  QuaternionUnits=off  OutputVector=[1]  ActiveIO=on  Width=1  DialogClass=MechanicalSensorBlock  Primitive=P1  Force=off  ForceUnits=N  Torque=off  TorqueUnits=N*m  ReferenceFrame=Absolute (World)  ReactionSensedSide=Base  ReactionReferenceFrame=Absolute (World)  ReactionForce=off  ReactionForceUnits=N  ReactionMoment=off  ReactionMomentUnits=N*m
  Memory : Memory
  Mux1 : Mux  Inputs=3
  Prismatic1 : mblibv1/Joints/Prismatic  LConnTagsString=__newl0|SA1  RConnTagsString=__newr0  UpdateFromCAD=off  NumSAPorts=1  CutJoint=off  MarkAsCut=off  Primitives=prismatic  PrimitiveProps=P1$World$[0 1 0]$prismatic  DialogClass=JointBlock  P1Axis=[0 1 0]
  Selector1 : Selector  InputPortWidth=3  IndexOptions=Index vector (dialog)  Indices=[2]  OutputSizes=1
  Selector2 : Selector  InputPortWidth=3  IndexOptions=Index vector (dialog)  Indices=[2]  OutputSizes=1
  Subsystem : Subsystem
  bar1 : mblibv1/Utilities/Mechanical Branching Bar  LConnTagsString=_newl0  RConnTagsString=SA0|SA1  UpdateFromCAD=off  DialogClass=MechanicalBranchingBarBlock  NumSAPorts=2
  bar2 : mblibv1/Utilities/Mechanical Branching Bar  LConnTagsString=_newl0  RConnTagsString=__newr0|SA2|SA3  UpdateFromCAD=off  DialogClass=MechanicalBranchingBarBlock  NumSAPorts=3
  pattern : Subsystem  mask{Amp=amp, Offset=0, freq=freq}
      mask prompts: Amp "Amplitude"; freq "Frequency"
      mask TypeOptions freq: Constant/Value
  "scope1 " : Scope
      settings: ShowLegends=on  SaveName=ScopeData11
  Conn1 : PMIOPort  Port=1  Side=Left
  force : Outport
  EE pos : Outport  Port=2
  leg length : Outport  Port=3
  wires:
  Mux1/1 -> Body Actuator/1
  Selector1/1 -> EE pos/1, Subsystem/1(pos)  "toe pos"
  Body Sensor/1 -> Selector2/1
  Joint Sensor/1 -> leg length/1
  Body Sensor1/1 -> Selector1/1
  Selector2/1 -> Subsystem/2(vel)
  Subsystem/1(force) -> Memory/1  "force"
  Constant/1 -> Mux1/1, Mux1/3
  df/1 -> pattern/1(df)
  pattern/1(PVA) -> "scope1 "/1, Joint Actuator/1
  Memory/1 -> Mux1/2, force/1
  connections:
  Conn1/RConn1 -- Prismatic1/LConn1
  bar2/LConn1 -- Body1/RConn1
  Prismatic1/RConn1 -- Body1/LConn1
  bar1/LConn1 -- Prismatic1/LConn2
  Joint Actuator/RConn1 -- bar1/RConn1
  bar1/RConn2 -- Joint Sensor/LConn1
  bar2/RConn1 -- Body Actuator/RConn1
  Body Sensor/LConn1 -- bar2/RConn3
  Body Sensor1/LConn1 -- bar2/RConn2

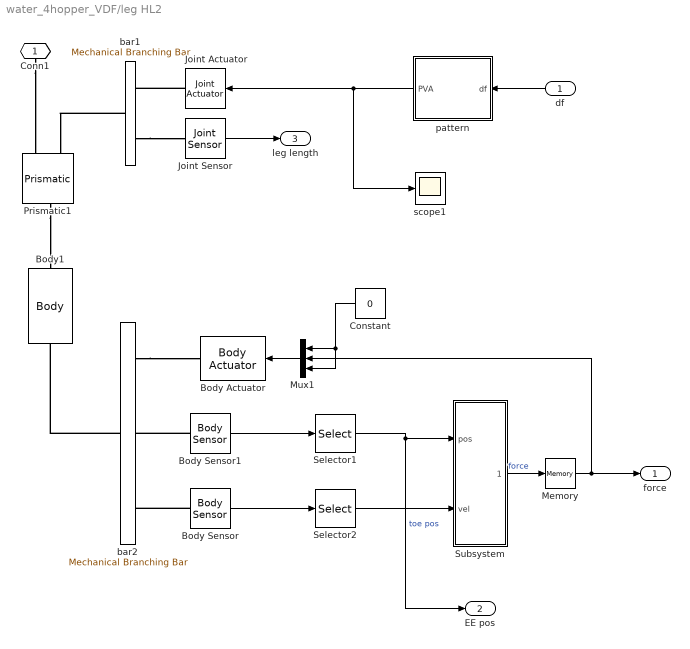
== system water_4hopper_VDF/leg HL2 ==
  df : Inport
  Body Actuator : mblibv1/Sensors &  Actuators/Body Actuator  UpdateFromCAD=off  PhysicalDomain=Mechanical  PortType=blob  ActuationStyle=Force  AngleUnits=deg  ArcVelocityUnits=deg/s  ArcAccelerationUnits=deg/s^2  CoordPositionUnits=m  VelocityUnits=m/s  AccelerationUnits=m/s^2  ForceUnits=N  TorqueUnits=N*m  ActiveIO=on  Width=3  DialogClass=MechanicalActuatorBlock  ReferenceFrame=Local (Body CS)  Angle=off  CoordPosition=on  Force=on  Torque=off
  Body Sensor : mblibv1/Sensors &  Actuators/Body Sensor  UpdateFromCAD=off  PhysicalDomain=Mechanical  PortType=blob  Muxed=on  Pose=off  Angle=on  AngleUnits=deg  ArcVelocity=off  ArcVelocityUnits=deg/s  ArcAcceleration=off  ArcAccelerationUnits=deg/s^2  CoordPosition=off  CoordPositionUnits=m  Velocity=on  VelocityUnits=m/s  Acceleration=off  AccelerationUnits=m/s^2  Quaternion=on  QuaternionDT=off  QuaternionDDT=off  QuaternionUnits=off  OutputVector=[1]  ActiveIO=on  Width=3  DialogClass=MechanicalSensorBlock  ReferenceFrame=Local (Body CS)
  Body Sensor1 : mblibv1/Sensors &  Actuators/Body Sensor  UpdateFromCAD=off  PhysicalDomain=Mechanical  PortType=blob  Muxed=on  Pose=off  Angle=on  AngleUnits=deg  ArcVelocity=off  ArcVelocityUnits=deg/s  ArcAcceleration=off  ArcAccelerationUnits=deg/s^2  CoordPosition=on  CoordPositionUnits=m  Velocity=off  VelocityUnits=m/s  Acceleration=off  AccelerationUnits=m/s^2  Quaternion=on  QuaternionDT=off  QuaternionDDT=off  QuaternionUnits=off  OutputVector=[1]  ActiveIO=on  Width=3  DialogClass=MechanicalSensorBlock  ReferenceFrame=Absolute (World)
  Body1 : mblibv1/Bodies/Body  LConnTagsString=CG  RConnTagsString=CS1  UpdateFromCAD=off  DialogClass=MechanicalBodyBlock  Mass=m_toe  MassUnits=kg  InertiaUnits=kg*m^2  Inertia=0.*eye(3)  Shape=Cylinder  ShapeDims=[1 1]  ShapeUnits=m  ShapeUse=false  Density=1  DensityUnits=kg/m^3  DensityUse=false  GraphicsMode=CONVHULL  BodyColorSelMode=MACHINE_DEFAULT  BodyColor=[1 0 0]  AttachedToCS=CG  CG=Left$CG$[0 0 0]$Adjoining$Adjoining$m$[0 0 0]$Euler X-Y-Z$deg$WORLD$true$none  WorkingFrames=Right$CS1$[0 -leg_length 0]$CG$CG$m$[0 0 0]$Euler X-Y-Z$deg$WORLD$true$none#Left$CS2$[0 0 0]$CG$CG$m$[0 0 0]$Euler X-Y-Z$deg$WORLD$false$none  CGPos=[0 0 0]  CGRot=[0 0 0]  CS0Pos=[]  CS0Rot=[]  CS1Pos=[0 -leg_length 0]  CS1Rot=[0 0 0]  CS2Pos=[0 0 0]  CS2Rot=[0 0 0]  CS3Pos=[]  CS3Rot=[]  CS4Pos=[]  CS4Rot=[]  CS5Pos=[]  CS5Rot=[]  CS6Pos=[]  CS6Rot=[]  CS7Pos=[]  CS7Rot=[]  CS8Pos=[]  CS8Rot=[]  CS9Pos=[]  CS9Rot=[]  CS10Pos=[]  CS10Rot=[]  CS11Pos=[]  CS11Rot=[]  CS12Pos=[]  CS12Rot=[]  CS13Pos=[]  CS13Rot=[]  CS14Pos=[]  CS14Rot=[]  CS15Pos=[]  CS15Rot=[]  CS16Pos=[]  CS16Rot=[]  CS17Pos=[]  CS17Rot=[]  CS18Pos=[]  CS18Rot=[]  CS19Pos=[]  CS19Rot=[]  CS20Pos=[]  CS20Rot=[]
  Constant : Constant  Value=0
  Joint Actuator : mblibv1/Sensors &  Actuators/Joint Actuator  UpdateFromCAD=off  PhysicalDomain=Mechanical  PortType=blob  ActuationStyle=Motion  AngleUnits=deg  ArcVelocityUnits=deg/s  ArcAccelerationUnits=deg/s^2  CoordPositionUnits=m  VelocityUnits=m/s  AccelerationUnits=m/s^2  ForceUnits=N  TorqueUnits=N*m  ActiveIO=on  Width=3  DialogClass=MechanicalActuatorBlock  Primitive=P1  ReferenceFrame=Absolute (World)
  Joint Sensor : mblibv1/Sensors &  Actuators/Joint Sensor  UpdateFromCAD=off  PhysicalDomain=Mechanical  PortType=blob  Muxed=on  Pose=off  Angle=on  AngleUnits=deg  ArcVelocity=off  ArcVelocityUnits=deg/s  ArcAcceleration=off  ArcAccelerationUnits=deg/s^2  CoordPosition=on  CoordPositionUnits=m  Velocity=off  VelocityUnits=m/s  Acceleration=off  AccelerationUnits=m/s^2  Quaternion=on  QuaternionDT=off  QuaternionDDT=off  QuaternionUnits=off  OutputVector=[1]  ActiveIO=on  Width=1  DialogClass=MechanicalSensorBlock  Primitive=P1  Force=off  ForceUnits=N  Torque=off  TorqueUnits=N*m  ReferenceFrame=Absolute (World)  ReactionSensedSide=Base  ReactionReferenceFrame=Absolute (World)  ReactionForce=off  ReactionForceUnits=N  ReactionMoment=off  ReactionMomentUnits=N*m
  Memory : Memory
  Mux1 : Mux  Inputs=3
  Prismatic1 : mblibv1/Joints/Prismatic  LConnTagsString=__newl0|SA1  RConnTagsString=__newr0  UpdateFromCAD=off  NumSAPorts=1  CutJoint=off  MarkAsCut=off  Primitives=prismatic  PrimitiveProps=P1$World$[0 1 0]$prismatic  DialogClass=JointBlock  P1Axis=[0 1 0]
  Selector1 : Selector  InputPortWidth=3  IndexOptions=Index vector (dialog)  Indices=[2]  OutputSizes=1
  Selector2 : Selector  InputPortWidth=3  IndexOptions=Index vector (dialog)  Indices=[2]  OutputSizes=1
  Subsystem : Subsystem
  bar1 : mblibv1/Utilities/Mechanical Branching Bar  LConnTagsString=_newl0  RConnTagsString=SA0|SA1  UpdateFromCAD=off  DialogClass=MechanicalBranchingBarBlock  NumSAPorts=2
  bar2 : mblibv1/Utilities/Mechanical Branching Bar  LConnTagsString=_newl0  RConnTagsString=__newr0|SA2|SA3  UpdateFromCAD=off  DialogClass=MechanicalBranchingBarBlock  NumSAPorts=3
  pattern : Subsystem  mask{Amp=amp, Offset=0, freq=freq}
      mask prompts: Amp "Amplitude"; freq "Frequency"
      mask TypeOptions freq: Constant/Value
  "scope1 " : Scope
      settings: ShowLegends=on  SaveName=ScopeData11
  Conn1 : PMIOPort  Port=1  Side=Left
  force : Outport
  EE pos : Outport  Port=2
  leg length : Outport  Port=3
  wires:
  Mux1/1 -> Body Actuator/1
  Selector1/1 -> EE pos/1, Subsystem/1(pos)  "toe pos"
  Body Sensor/1 -> Selector2/1
  Joint Sensor/1 -> leg length/1
  Body Sensor1/1 -> Selector1/1
  Selector2/1 -> Subsystem/2(vel)
  Subsystem/1(force) -> Memory/1  "force"
  Constant/1 -> Mux1/1, Mux1/3
  df/1 -> pattern/1(df)
  pattern/1(PVA) -> "scope1 "/1, Joint Actuator/1
  Memory/1 -> Mux1/2, force/1
  connections:
  Conn1/RConn1 -- Prismatic1/LConn1
  bar2/LConn1 -- Body1/RConn1
  Prismatic1/RConn1 -- Body1/LConn1
  bar1/LConn1 -- Prismatic1/LConn2
  Joint Actuator/RConn1 -- bar1/RConn1
  bar1/RConn2 -- Joint Sensor/LConn1
  bar2/RConn1 -- Body Actuator/RConn1
  Body Sensor/LConn1 -- bar2/RConn3
  Body Sensor1/LConn1 -- bar2/RConn2

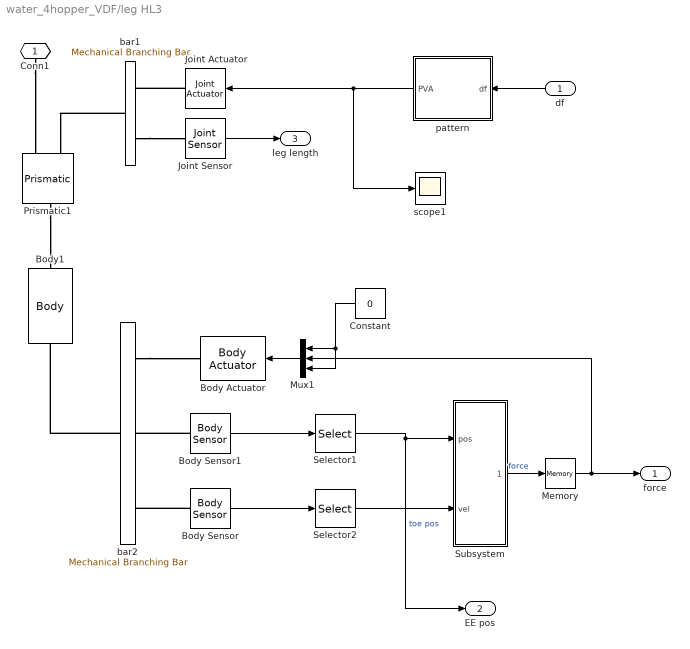
== system water_4hopper_VDF/leg HL3 ==
  df : Inport
  Body Actuator : mblibv1/Sensors &  Actuators/Body Actuator  UpdateFromCAD=off  PhysicalDomain=Mechanical  PortType=blob  ActuationStyle=Force  AngleUnits=deg  ArcVelocityUnits=deg/s  ArcAccelerationUnits=deg/s^2  CoordPositionUnits=m  VelocityUnits=m/s  AccelerationUnits=m/s^2  ForceUnits=N  TorqueUnits=N*m  ActiveIO=on  Width=3  DialogClass=MechanicalActuatorBlock  ReferenceFrame=Local (Body CS)  Angle=off  CoordPosition=on  Force=on  Torque=off
  Body Sensor : mblibv1/Sensors &  Actuators/Body Sensor  UpdateFromCAD=off  PhysicalDomain=Mechanical  PortType=blob  Muxed=on  Pose=off  Angle=on  AngleUnits=deg  ArcVelocity=off  ArcVelocityUnits=deg/s  ArcAcceleration=off  ArcAccelerationUnits=deg/s^2  CoordPosition=off  CoordPositionUnits=m  Velocity=on  VelocityUnits=m/s  Acceleration=off  AccelerationUnits=m/s^2  Quaternion=on  QuaternionDT=off  QuaternionDDT=off  QuaternionUnits=off  OutputVector=[1]  ActiveIO=on  Width=3  DialogClass=MechanicalSensorBlock  ReferenceFrame=Local (Body CS)
  Body Sensor1 : mblibv1/Sensors &  Actuators/Body Sensor  UpdateFromCAD=off  PhysicalDomain=Mechanical  PortType=blob  Muxed=on  Pose=off  Angle=on  AngleUnits=deg  ArcVelocity=off  ArcVelocityUnits=deg/s  ArcAcceleration=off  ArcAccelerationUnits=deg/s^2  CoordPosition=on  CoordPositionUnits=m  Velocity=off  VelocityUnits=m/s  Acceleration=off  AccelerationUnits=m/s^2  Quaternion=on  QuaternionDT=off  QuaternionDDT=off  QuaternionUnits=off  OutputVector=[1]  ActiveIO=on  Width=3  DialogClass=MechanicalSensorBlock  ReferenceFrame=Absolute (World)
  Body1 : mblibv1/Bodies/Body  LConnTagsString=CG  RConnTagsString=CS1  UpdateFromCAD=off  DialogClass=MechanicalBodyBlock  Mass=m_toe  MassUnits=kg  InertiaUnits=kg*m^2  Inertia=0.*eye(3)  Shape=Cylinder  ShapeDims=[1 1]  ShapeUnits=m  ShapeUse=false  Density=1  DensityUnits=kg/m^3  DensityUse=false  GraphicsMode=CONVHULL  BodyColorSelMode=MACHINE_DEFAULT  BodyColor=[1 0 0]  AttachedToCS=CG  CG=Left$CG$[0 0 0]$Adjoining$Adjoining$m$[0 0 0]$Euler X-Y-Z$deg$WORLD$true$none  WorkingFrames=Right$CS1$[0 -leg_length 0]$CG$CG$m$[0 0 0]$Euler X-Y-Z$deg$WORLD$true$none#Left$CS2$[0 0 0]$CG$CG$m$[0 0 0]$Euler X-Y-Z$deg$WORLD$false$none  CGPos=[0 0 0]  CGRot=[0 0 0]  CS0Pos=[]  CS0Rot=[]  CS1Pos=[0 -leg_length 0]  CS1Rot=[0 0 0]  CS2Pos=[0 0 0]  CS2Rot=[0 0 0]  CS3Pos=[]  CS3Rot=[]  CS4Pos=[]  CS4Rot=[]  CS5Pos=[]  CS5Rot=[]  CS6Pos=[]  CS6Rot=[]  CS7Pos=[]  CS7Rot=[]  CS8Pos=[]  CS8Rot=[]  CS9Pos=[]  CS9Rot=[]  CS10Pos=[]  CS10Rot=[]  CS11Pos=[]  CS11Rot=[]  CS12Pos=[]  CS12Rot=[]  CS13Pos=[]  CS13Rot=[]  CS14Pos=[]  CS14Rot=[]  CS15Pos=[]  CS15Rot=[]  CS16Pos=[]  CS16Rot=[]  CS17Pos=[]  CS17Rot=[]  CS18Pos=[]  CS18Rot=[]  CS19Pos=[]  CS19Rot=[]  CS20Pos=[]  CS20Rot=[]
  Constant : Constant  Value=0
  Joint Actuator : mblibv1/Sensors &  Actuators/Joint Actuator  UpdateFromCAD=off  PhysicalDomain=Mechanical  PortType=blob  ActuationStyle=Motion  AngleUnits=deg  ArcVelocityUnits=deg/s  ArcAccelerationUnits=deg/s^2  CoordPositionUnits=m  VelocityUnits=m/s  AccelerationUnits=m/s^2  ForceUnits=N  TorqueUnits=N*m  ActiveIO=on  Width=3  DialogClass=MechanicalActuatorBlock  Primitive=P1  ReferenceFrame=Absolute (World)
  Joint Sensor : mblibv1/Sensors &  Actuators/Joint Sensor  UpdateFromCAD=off  PhysicalDomain=Mechanical  PortType=blob  Muxed=on  Pose=off  Angle=on  AngleUnits=deg  ArcVelocity=off  ArcVelocityUnits=deg/s  ArcAcceleration=off  ArcAccelerationUnits=deg/s^2  CoordPosition=on  CoordPositionUnits=m  Velocity=off  VelocityUnits=m/s  Acceleration=off  AccelerationUnits=m/s^2  Quaternion=on  QuaternionDT=off  QuaternionDDT=off  QuaternionUnits=off  OutputVector=[1]  ActiveIO=on  Width=1  DialogClass=MechanicalSensorBlock  Primitive=P1  Force=off  ForceUnits=N  Torque=off  TorqueUnits=N*m  ReferenceFrame=Absolute (World)  ReactionSensedSide=Base  ReactionReferenceFrame=Absolute (World)  ReactionForce=off  ReactionForceUnits=N  ReactionMoment=off  ReactionMomentUnits=N*m
  Memory : Memory
  Mux1 : Mux  Inputs=3
  Prismatic1 : mblibv1/Joints/Prismatic  LConnTagsString=__newl0|SA1  RConnTagsString=__newr0  UpdateFromCAD=off  NumSAPorts=1  CutJoint=off  MarkAsCut=off  Primitives=prismatic  PrimitiveProps=P1$World$[0 1 0]$prismatic  DialogClass=JointBlock  P1Axis=[0 1 0]
  Selector1 : Selector  InputPortWidth=3  IndexOptions=Index vector (dialog)  Indices=[2]  OutputSizes=1
  Selector2 : Selector  InputPortWidth=3  IndexOptions=Index vector (dialog)  Indices=[2]  OutputSizes=1
  Subsystem : Subsystem
  bar1 : mblibv1/Utilities/Mechanical Branching Bar  LConnTagsString=_newl0  RConnTagsString=SA0|SA1  UpdateFromCAD=off  DialogClass=MechanicalBranchingBarBlock  NumSAPorts=2
  bar2 : mblibv1/Utilities/Mechanical Branching Bar  LConnTagsString=_newl0  RConnTagsString=__newr0|SA2|SA3  UpdateFromCAD=off  DialogClass=MechanicalBranchingBarBlock  NumSAPorts=3
  pattern : Subsystem  mask{Amp=amp, Offset=0, freq=freq}
      mask prompts: Amp "Amplitude"; freq "Frequency"
      mask TypeOptions freq: Constant/Value
  "scope1 " : Scope
      settings: ShowLegends=on  SaveName=ScopeData11
  Conn1 : PMIOPort  Port=1  Side=Left
  force : Outport
  EE pos : Outport  Port=2
  leg length : Outport  Port=3
  wires:
  Mux1/1 -> Body Actuator/1
  Selector1/1 -> EE pos/1, Subsystem/1(pos)  "toe pos"
  Body Sensor/1 -> Selector2/1
  Joint Sensor/1 -> leg length/1
  Body Sensor1/1 -> Selector1/1
  Selector2/1 -> Subsystem/2(vel)
  Subsystem/1(force) -> Memory/1  "force"
  Constant/1 -> Mux1/1, Mux1/3
  df/1 -> pattern/1(df)
  pattern/1(PVA) -> "scope1 "/1, Joint Actuator/1
  Memory/1 -> Mux1/2, force/1
  connections:
  Conn1/RConn1 -- Prismatic1/LConn1
  bar2/LConn1 -- Body1/RConn1
  Prismatic1/RConn1 -- Body1/LConn1
  bar1/LConn1 -- Prismatic1/LConn2
  Joint Actuator/RConn1 -- bar1/RConn1
  bar1/RConn2 -- Joint Sensor/LConn1
  bar2/RConn1 -- Body Actuator/RConn1
  Body Sensor/LConn1 -- bar2/RConn3
  Body Sensor1/LConn1 -- bar2/RConn2

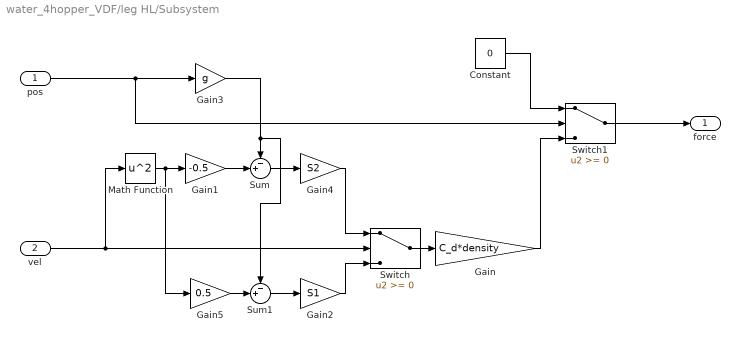
== system water_4hopper_VDF/leg HL/Subsystem ==
  pos : Inport
  vel : Inport  Port=2
  Constant : Constant  Value=0
  Gain : Gain  Gain=C_d*density
  Gain1 : Gain  Gain=-0.5
  Gain2 : Gain  Gain=S1
  Gain3 : Gain  Gain=g
  Gain4 : Gain  Gain=S2
  Gain5 : Gain  Gain=0.5
  Math Function : Math  Operator=square  SaturateOnIntegerOverflow=on
  Sum : Sum  Inputs=-+|
  Sum1 : Sum  Inputs=-+|
  Switch : Switch  ZeroCross=off
  Switch1 : Switch
  force : Outport
  wires:
  Gain5/1 -> Sum1/2
  Sum1/1 -> Gain2/1
  Constant/1 -> Switch1/1
  Gain/1 -> Switch1/3
  Switch1/1 -> force/1
  Switch/1 -> Gain/1
  Gain2/1 -> Switch/3
  Gain4/1 -> Switch/1
  Sum/1 -> Gain4/1
  Gain3/1 -> Sum1/1, Sum/1
  pos/1 -> Switch1/2, Gain3/1
  Gain1/1 -> Sum/2
  Math Function/1 -> Gain5/1, Gain1/1
  vel/1 -> Math Function/1, Switch/2

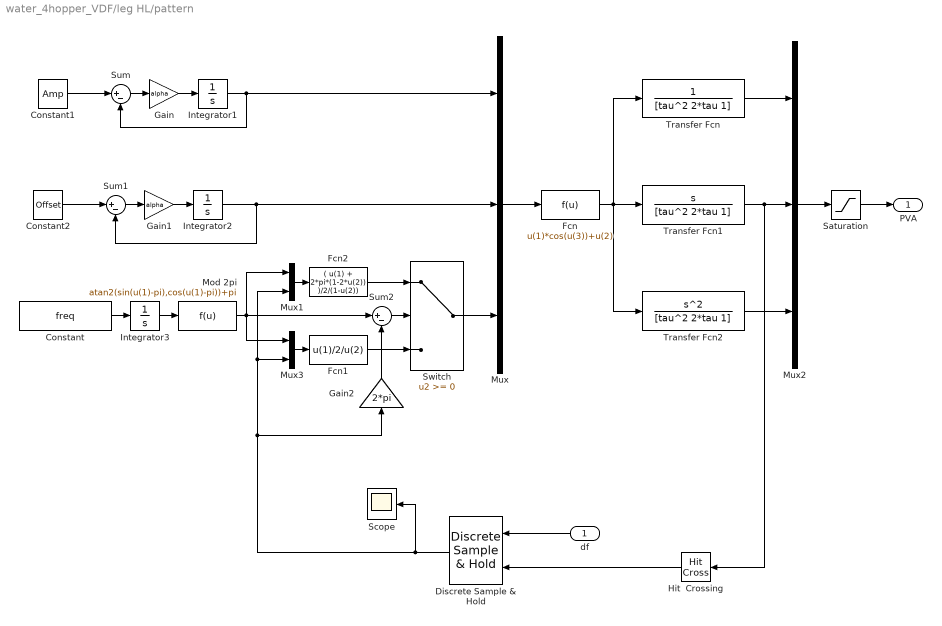
== system water_4hopper_VDF/leg HL/pattern ==
  df : Inport
  Constant : Constant  Value=freq
  Constant1 : Constant  Value=Amp
  Constant2 : Constant  Value=Offset
  Discrete Sample & Hold : powerlib_extras/Discrete  Control Blocks/Discrete Sample & Hold  ic=0.5  Ts=2/pi/freq/20
  Fcn : Fcn  Expr=u(1)*cos(u(3))+u(2)
  Fcn1 : Fcn  Expr=u(1)/2/u(2)
  Fcn2 : Fcn  Expr=( u(1) + 2*pi*(1-2*u(2)) )/2/(1-u(2))
  Gain : Gain  Gain=alpha
  Gain1 : Gain  Gain=alpha
  Gain2 : Gain  Gain=2*pi
  Hit  Crossing : HitCross  HitCrossingDirection=falling
  Integrator1 : Integrator
  Integrator2 : Integrator
  Integrator3 : Integrator  InitialCondition=0.001*rand
  Mod 2pi : Fcn  Expr=atan2(sin(u(1)-pi),cos(u(1)-pi))+pi
  Mux : Mux  Inputs=3
  Mux1 : Mux  Inputs=2
  Mux2 : Mux  Inputs=3
  Mux3 : Mux  Inputs=2
  Saturation : Saturate  UpperLimit=3*amp*freq^2  LowerLimit=-3*amp*freq^2
  Scope : Scope
  Sum : Sum  Inputs=|+-
  Sum1 : Sum  Inputs=|+-
  Sum2 : Sum  Inputs=|+-
  Switch : Switch
  Transfer Fcn : TransferFcn  Denominator=[tau^2 2*tau 1]
  Transfer Fcn1 : TransferFcn  Numerator=[1 0]  Denominator=[tau^2 2*tau 1]
  Transfer Fcn2 : TransferFcn  Numerator=[1 0 0]  Denominator=[tau^2 2*tau 1]
  PVA : Outport
  wires:
  Constant/1 -> Integrator3/1
  Mod 2pi/1 -> Mux1/1, Mux3/1, Sum2/1
  Integrator3/1 -> Mod 2pi/1
  Switch/1 -> Mux/3
  Fcn1/1 -> Switch/3
  Fcn2/1 -> Switch/1
  Mux/1 -> Fcn/1
  Gain1/1 -> Integrator2/1
  Constant2/1 -> Sum1/1
  Integrator2/1 -> Mux/2, Sum1/2
  Sum1/1 -> Gain1/1
  Gain/1 -> Integrator1/1
  Constant1/1 -> Sum/1
  Integrator1/1 -> Mux/1, Sum/2
  Sum/1 -> Gain/1
  Transfer Fcn2/1 -> Mux2/3
  Transfer Fcn/1 -> Mux2/1
  Transfer Fcn1/1 -> Hit  Crossing/1, Mux2/2
  Mux2/1 -> Saturation/1
  Fcn/1 -> Transfer Fcn1/1, Transfer Fcn/1, Transfer Fcn2/1
  Saturation/1 -> PVA/1
  Hit  Crossing/1 -> Discrete Sample & Hold/2
  Sum2/1 -> Switch/2
  Gain2/1 -> Sum2/2
  Discrete Sample & Hold/1 -> Scope/1, Mux3/2, Mux1/2, Gain2/1
  Mux1/1 -> Fcn2/1
  Mux3/1 -> Fcn1/1
  df/1 -> Discrete Sample & Hold/1

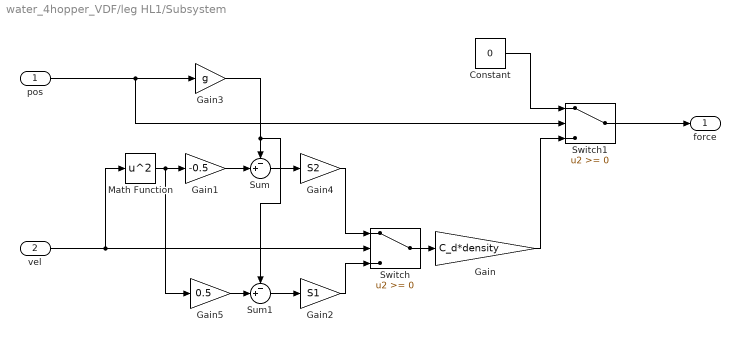
== system water_4hopper_VDF/leg HL1/Subsystem ==
  pos : Inport
  vel : Inport  Port=2
  Constant : Constant  Value=0
  Gain : Gain  Gain=C_d*density
  Gain1 : Gain  Gain=-0.5
  Gain2 : Gain  Gain=S1
  Gain3 : Gain  Gain=g
  Gain4 : Gain  Gain=S2
  Gain5 : Gain  Gain=0.5
  Math Function : Math  Operator=square  SaturateOnIntegerOverflow=on
  Sum : Sum  Inputs=-+|
  Sum1 : Sum  Inputs=-+|
  Switch : Switch  ZeroCross=off
  Switch1 : Switch
  force : Outport
  wires:
  Gain5/1 -> Sum1/2
  Sum1/1 -> Gain2/1
  Constant/1 -> Switch1/1
  Gain/1 -> Switch1/3
  Switch1/1 -> force/1
  Switch/1 -> Gain/1
  Gain2/1 -> Switch/3
  Gain4/1 -> Switch/1
  Sum/1 -> Gain4/1
  Gain3/1 -> Sum1/1, Sum/1
  pos/1 -> Switch1/2, Gain3/1
  Gain1/1 -> Sum/2
  Math Function/1 -> Gain5/1, Gain1/1
  vel/1 -> Math Function/1, Switch/2

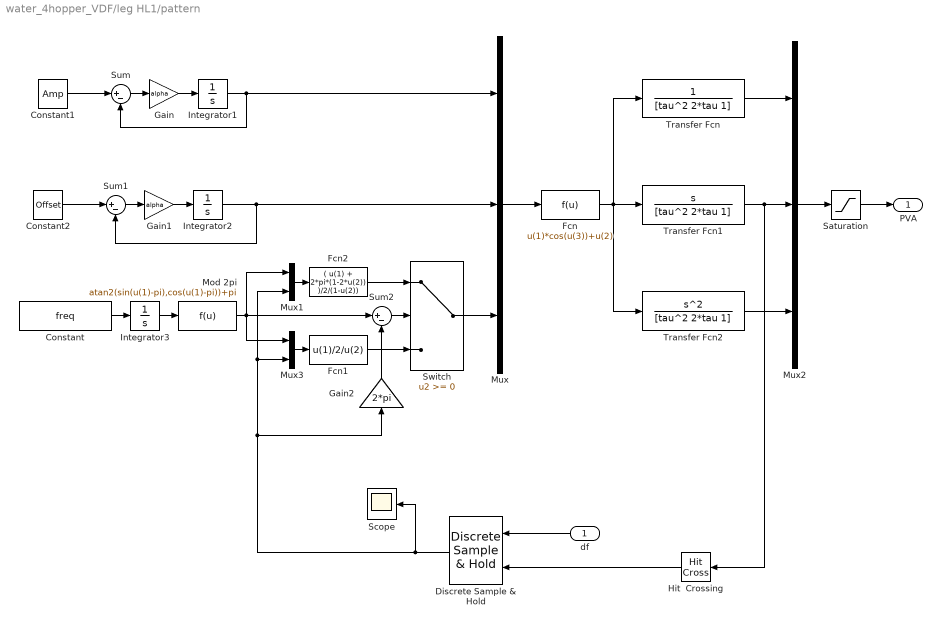
== system water_4hopper_VDF/leg HL1/pattern ==
  df : Inport
  Constant : Constant  Value=freq
  Constant1 : Constant  Value=Amp
  Constant2 : Constant  Value=Offset
  Discrete Sample & Hold : powerlib_extras/Discrete  Control Blocks/Discrete Sample & Hold  ic=0.5  Ts=2/pi/freq/20
  Fcn : Fcn  Expr=u(1)*cos(u(3))+u(2)
  Fcn1 : Fcn  Expr=u(1)/2/u(2)
  Fcn2 : Fcn  Expr=( u(1) + 2*pi*(1-2*u(2)) )/2/(1-u(2))
  Gain : Gain  Gain=alpha
  Gain1 : Gain  Gain=alpha
  Gain2 : Gain  Gain=2*pi
  Hit  Crossing : HitCross  HitCrossingDirection=falling
  Integrator1 : Integrator
  Integrator2 : Integrator
  Integrator3 : Integrator  InitialCondition=0.001*rand
  Mod 2pi : Fcn  Expr=atan2(sin(u(1)-pi),cos(u(1)-pi))+pi
  Mux : Mux  Inputs=3
  Mux1 : Mux  Inputs=2
  Mux2 : Mux  Inputs=3
  Mux3 : Mux  Inputs=2
  Saturation : Saturate  UpperLimit=3*amp*freq^2  LowerLimit=-3*amp*freq^2
  Scope : Scope
  Sum : Sum  Inputs=|+-
  Sum1 : Sum  Inputs=|+-
  Sum2 : Sum  Inputs=|+-
  Switch : Switch
  Transfer Fcn : TransferFcn  Denominator=[tau^2 2*tau 1]
  Transfer Fcn1 : TransferFcn  Numerator=[1 0]  Denominator=[tau^2 2*tau 1]
  Transfer Fcn2 : TransferFcn  Numerator=[1 0 0]  Denominator=[tau^2 2*tau 1]
  PVA : Outport
  wires:
  Constant/1 -> Integrator3/1
  Mod 2pi/1 -> Mux1/1, Mux3/1, Sum2/1
  Integrator3/1 -> Mod 2pi/1
  Switch/1 -> Mux/3
  Fcn1/1 -> Switch/3
  Fcn2/1 -> Switch/1
  Mux/1 -> Fcn/1
  Gain1/1 -> Integrator2/1
  Constant2/1 -> Sum1/1
  Integrator2/1 -> Mux/2, Sum1/2
  Sum1/1 -> Gain1/1
  Gain/1 -> Integrator1/1
  Constant1/1 -> Sum/1
  Integrator1/1 -> Mux/1, Sum/2
  Sum/1 -> Gain/1
  Transfer Fcn2/1 -> Mux2/3
  Transfer Fcn/1 -> Mux2/1
  Transfer Fcn1/1 -> Hit  Crossing/1, Mux2/2
  Mux2/1 -> Saturation/1
  Fcn/1 -> Transfer Fcn1/1, Transfer Fcn/1, Transfer Fcn2/1
  Saturation/1 -> PVA/1
  Hit  Crossing/1 -> Discrete Sample & Hold/2
  Sum2/1 -> Switch/2
  Gain2/1 -> Sum2/2
  Discrete Sample & Hold/1 -> Scope/1, Mux3/2, Mux1/2, Gain2/1
  Mux1/1 -> Fcn2/1
  Mux3/1 -> Fcn1/1
  df/1 -> Discrete Sample & Hold/1

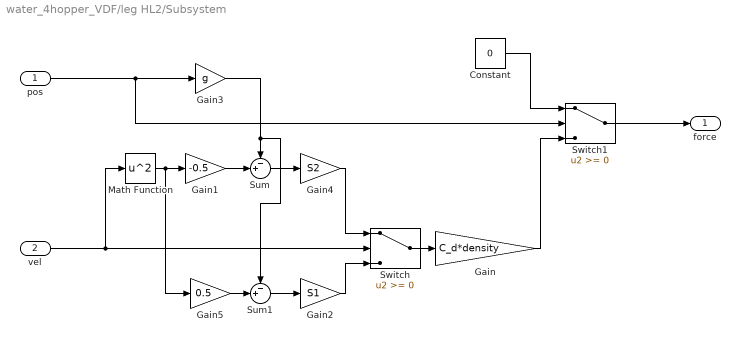
== system water_4hopper_VDF/leg HL2/Subsystem ==
  pos : Inport
  vel : Inport  Port=2
  Constant : Constant  Value=0
  Gain : Gain  Gain=C_d*density
  Gain1 : Gain  Gain=-0.5
  Gain2 : Gain  Gain=S1
  Gain3 : Gain  Gain=g
  Gain4 : Gain  Gain=S2
  Gain5 : Gain  Gain=0.5
  Math Function : Math  Operator=square  SaturateOnIntegerOverflow=on
  Sum : Sum  Inputs=-+|
  Sum1 : Sum  Inputs=-+|
  Switch : Switch  ZeroCross=off
  Switch1 : Switch
  force : Outport
  wires:
  Gain5/1 -> Sum1/2
  Sum1/1 -> Gain2/1
  Constant/1 -> Switch1/1
  Gain/1 -> Switch1/3
  Switch1/1 -> force/1
  Switch/1 -> Gain/1
  Gain2/1 -> Switch/3
  Gain4/1 -> Switch/1
  Sum/1 -> Gain4/1
  Gain3/1 -> Sum1/1, Sum/1
  pos/1 -> Switch1/2, Gain3/1
  Gain1/1 -> Sum/2
  Math Function/1 -> Gain5/1, Gain1/1
  vel/1 -> Math Function/1, Switch/2
